simulink library "MPC_51_v6_GP_CL"  (R2020a)
settings: Solver=VariableStepAuto  StartTime=0.0  StopTime=10.0  RelTol=1e-3
libraries: MPC_Sublibraries x4
settings Model: Creator=John Jr  LastModifiedBy=John Jr
settings DataIOCC: ReturnWorkspaceOutputs=off
settings DebuggingCC: ArithmeticOperatorsInVariantConditions=warning
settings SFSimCC: CustomCodeUndefinedFunction=UseInterfaceOnly

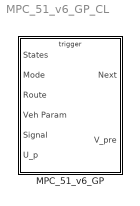
== system MPC_51_v6_GP_CL ==
  MPC_51_v6_GP : Subsystem  TreatAsAtomicUnit=on
      mask Display:
      | patch([0 1 1 0], [0 0 1 1],[1 .8 1])
      | 
      | port_label('input',1,'\fontname{Cambria Math}States','texmode','on')
      | port_label('input',2,'\fontname{Cambria Math}Mode','texmode','on')
      | port_label('input',3,'\fontname{Cambria Math}Route','texmode','on')
      | port_label('input',4,'\fontname{Cambria Math}Param','texmode','on')
      | port_label('input',5,'\fontname{Cambria Math}Signal','texmode','on')
      | port_label('input',6,'\fontname{Cambria Math}T_{prev}','texmode','on')
      | 
      | port_label('output',1,'\fontname{Cambria Math}V_{MPC},T_{MPC}','texmode','on')
      | port_label('output',2,'\fontname{Cambria Math}V_{des}(1)','texmode','on')
      | 
      | port_label('trigger','\spadesuit','texmode','on')
      | 
      | disp('\fontname{Cambria Math}\fontsize{12}  MPC v6\newline  51 Step','texmode','on')

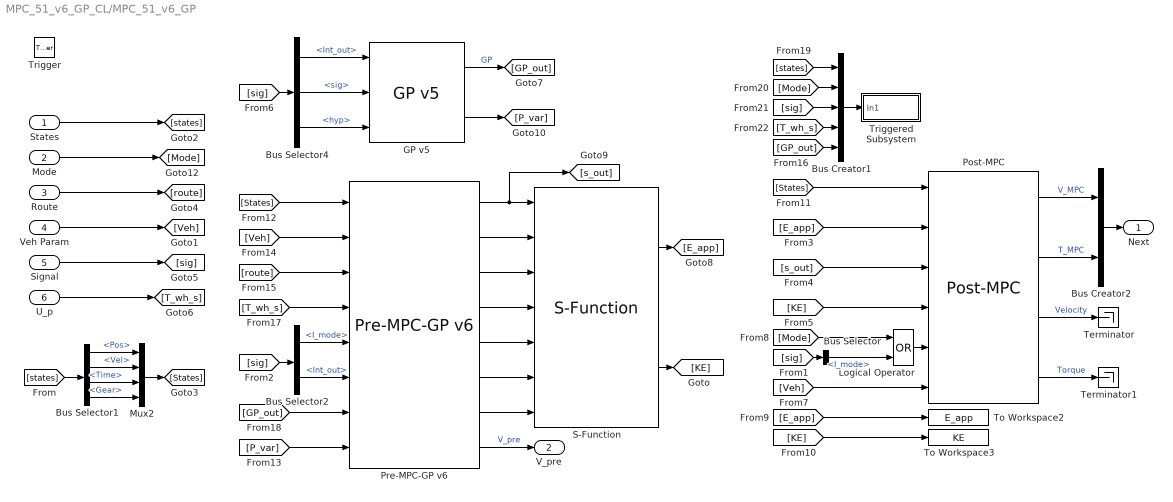
== system MPC_51_v6_GP_CL/MPC_51_v6_GP ==
  States : Inport
  Mode : Inport  Port=2
  Route : Inport  Port=3
  Veh Param : Inport  Port=4
  Signal : Inport  Port=5
  U_p : Inport  Port=6
  Trigger : TriggerPort  TriggerType=falling  VariantControl=Variant
  Bus Creator1 : BusCreator  Inputs=5
  Bus Creator2 : BusCreator  Inputs=2
  Bus Selector : BusSelector  OutputSignals=Signal.I_mode
  Bus Selector1 : BusSelector  OutputSignals=Pos,Vel,Time,Gear
  Bus Selector2 : BusSelector  OutputSignals=I_mode,Int_out
  Bus Selector4 : BusSelector  OutputSignals=Int_out,sig,hyp
  GP v5 : MPC_Sublibraries/GP v5  SystemSampleTime=-1  Latency=0  AutoFrameSizeCalculation=off
  Logical Operator : Logic  Operator=OR  AllPortsSameDT=off  OutDataTypeStr=boolean
  Mux2 : Mux
  Post-MPC : MPC_Sublibraries/Post-MPC  SystemSampleTime=-1  Latency=0  AutoFrameSizeCalculation=off
  Pre-MPC-GP v6 : MPC_Sublibraries/Pre-MPC-GP v6  SystemSampleTime=-1  Latency=0  AutoFrameSizeCalculation=off
  S-Function : MPC_Sublibraries/S-Function  SFunctionModules=solver_51_v2_wrapper
  Terminator : Terminator
  Terminator1 : Terminator
  To Workspace2 : ToWorkspace  VariableName=E_app  SampleTime=-1
  To Workspace3 : ToWorkspace  VariableName=KE  SampleTime=-1
  Triggered Subsystem : Subsystem  TreatAsAtomicUnit=on
      mask Display:
      | patch([0 1 1 0], [0 0 1 1],[.8 1 .8])
      | 
      | port_label('input',1,'MPC input')
  Next : Outport  VectorParamsAs1DForOutWhenUnconnected=off
  V_pre : Outport  Port=2  VectorParamsAs1DForOutWhenUnconnected=off
  wires:
  Bus Selector/1 -> Logical Operator/2  "<I_mode>"
  [sig] -> Bus Selector/1
  [Mode] -> Logical Operator/1
  States/1 -> [states]
  Route/1 -> [route]
  Bus Selector1/4 -> Mux2/4  "<Gear>"
  Bus Selector1/2 -> Mux2/2  "<Vel>"
  Bus Selector1/3 -> Mux2/3  "<Time>"
  Bus Selector1/1 -> Mux2/1  "<Pos>"
  [states] -> Bus Selector1/1
  Veh Param/1 -> [Veh]
  [Veh] -> Post-MPC/6
  Post-MPC/4 -> Terminator1/1  "Torque"
  Post-MPC/3 -> Terminator/1  "Velocity"
  Mux2/1 -> [States]
  [States] -> Post-MPC/1
  Mode/1 -> [Mode]
  [E_app] -> Post-MPC/2
  [s_out] -> Post-MPC/3
  [KE] -> Post-MPC/4
  Logical Operator/1 -> Post-MPC/5
  S-Function/2 -> [KE]
  S-Function/1 -> [E_app]
  Bus Creator2/1 -> Next/1
  Post-MPC/1 -> Bus Creator2/1  "V_MPC"
  Post-MPC/2 -> Bus Creator2/2  "T_MPC"
  Signal/1 -> [sig]
  [states] -> Bus Creator1/1
  [sig] -> Bus Creator1/3
  [T_wh_s] -> Bus Creator1/4
  Bus Creator1/1 -> Triggered Subsystem/1(In1)
  [Mode] -> Bus Creator1/2
  [GP_out] -> Bus Creator1/5
  [KE] -> To Workspace3/1
  [E_app] -> To Workspace2/1
  [T_wh_s] -> Pre-MPC-GP v6/4
  [route] -> Pre-MPC-GP v6/3
  [Veh] -> Pre-MPC-GP v6/2
  Bus Selector2/2 -> Pre-MPC-GP v6/6  "<Int_out>"
  [GP_out] -> Pre-MPC-GP v6/7
  Bus Selector2/1 -> Pre-MPC-GP v6/5  "<I_mode>"
  [States] -> Pre-MPC-GP v6/1
  [sig] -> Bus Selector2/1
  Pre-MPC-GP v6/1 -> S-Function/1, [s_out]
  Pre-MPC-GP v6/2 -> S-Function/2
  Pre-MPC-GP v6/3 -> S-Function/3
  Pre-MPC-GP v6/4 -> S-Function/4
  Pre-MPC-GP v6/5 -> S-Function/5
  Pre-MPC-GP v6/6 -> S-Function/6
  Pre-MPC-GP v6/7 -> S-Function/7
  Pre-MPC-GP v6/8 -> V_pre/1  "V_pre"
  U_p/1 -> [T_wh_s]
  Bus Selector4/3 -> GP v5/3  "<hyp>"
  GP v5/1 -> [GP_out]  "GP"
  Bus Selector4/1 -> GP v5/1  "<Int_out>"
  [sig] -> Bus Selector4/1
  Bus Selector4/2 -> GP v5/2  "<sig>"
  GP v5/2 -> [P_var]
  [P_var] -> Pre-MPC-GP v6/8

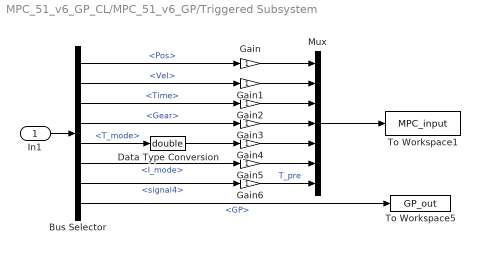
== system MPC_51_v6_GP_CL/MPC_51_v6_GP/Triggered Subsystem ==
  In1 : Inport
  Bus Selector : BusSelector  OutputSignals=signal1.Pos,signal1.Vel,signal1.Time,signal1.Gear,signal2.T_mode,signal3.I_mode,signal4,GP
  Data Type Conversion : DataTypeConversion  OutDataTypeStr=double
  Gain{,1..6} (7 alike) : Gain
  Mux : Mux  Inputs=7
  To Workspace1 : ToWorkspace  VariableName=MPC_input  SaveFormat=Structure With Time  SampleTime=-1
  To Workspace5 : ToWorkspace  VariableName=GP_out  SampleTime=-1
  wires:
  In1/1 -> Bus Selector/1
  Bus Selector/1 -> Gain/1  "<Pos>"
  Bus Selector/6 -> Gain5/1  "<I_mode>"
  Bus Selector/5 -> Data Type Conversion/1  "<T_mode>"
  Bus Selector/4 -> Gain3/1  "<Gear>"
  Bus Selector/3 -> Gain2/1  "<Time>"
  Bus Selector/2 -> Gain1/1  "<Vel>"
  Bus Selector/7 -> Gain6/1  "<signal4>"
  Gain6/1 -> Mux/7  "T_pre"
  Gain5/1 -> Mux/6
  Gain4/1 -> Mux/5
  Gain3/1 -> Mux/4
  Gain2/1 -> Mux/3
  Gain1/1 -> Mux/2
  Gain/1 -> Mux/1
  Mux/1 -> To Workspace1/1
  Data Type Conversion/1 -> Gain4/1
  Bus Selector/8 -> To Workspace5/1  "<GP>"
